simulink subsystem "ElectricalThermalSystemSSC"  (R2025b)
settings: Solver=VariableStepAuto  StartTime=0.0  StopTime=10.0  RelTol=1e-3
undefined symbols (not defined in the file): coolant_pipe_D, coolant_valve_D_ratio_max, coolant_valve_D_ratio_min, coolant_valve_displacement, EnvAirTemp, EnvGrvty, PlantThrEstCmpPwr, PlntThrChArea, PlntThrFanMaxSpd, PlntThrFanMechEff, PlntThrFanVolEff, PlntThrHeaterMaxPwr, PlntThrPipeArea, PlntThrPipeDia, PlntThrPmpMaxSpd, PlntThrRadRamEff, PlntThrRefrigAinit, PlntThrTankArea, PlntThrTankVol, PlntThrValDisp, PlntThrValDratioMax, PlntThrValDratioMin, PlntThrValSplMax, ThrmEM1, ThrmEM2, ThrmEM3, ThrmEM4
libraries: fl_lib x159, nesl_utility x69, SimscapeFluids_lib x25, autolibutils x12
(part 3 of 5)

== system ElectricalThermalSystemSSC/Battery/SC2 ==
  Absolute Reference (TL) : fl_lib/Thermal Liquid/Elements/Absolute Reference (TL)
  Mass & Energy Flow Rate Sensor (TL) : fl_lib/Thermal Liquid/Sensors/Flow Rate Sensor (TL)  mass_flow_measure=true  volumetric_flow_measure=false  energy_flow_measure=true
      settings: InternalSimscapePortConfiguration="{\"Bottom\":[{\"id\":\"PHI\",\"label\":\"φ\",\"type\":\"output\"}],\"Left\":[{\"id\":\"A\",\"label\":\"A\",\"type\":\"foundation.thermal_liquid.thermal_liquid\"}],\"Right\":[{\"id\":\"B\",\"label\":\"B\",\"type\":\"foundation.thermal_liquid.thermal_liquid\"},{\"id\":\"M\",\"label\":\"M\",\"type\":\"output\"}],\"Top\":[]}"
  PS-Simulink Converter : nesl_utility/PS-Simulink Converter  PhysicalDomain=network_engine_domain  SubClassName=ps_output  LeftPortType=input  RightPortType=output  PseudoPeriodic=off  Frequencies=[]  VectorFormat=1-D array  Unit=kg/s  AffineConversion=off
  Pressure & Temperature Sensor (TL) : fl_lib/Thermal Liquid/Sensors/Pressure & Temperature Sensor (TL)  reference=foundation.enum.MeasurementReference.difference  pressure=true  pressure_spec=foundation.enum.PressureMeasementSpec.Absolute  temperature=true
      settings: InternalSimscapePortConfiguration="{\"Bottom\":[{\"id\":\"T\",\"label\":\"T\",\"type\":\"output\"}],\"Left\":[{\"id\":\"A\",\"label\":\"A\",\"type\":\"foundation.thermal_liquid.thermal_liquid\"}],\"Right\":[{\"id\":\"B\",\"label\":\"B\",\"type\":\"foundation.thermal_liquid.thermal_liquid\"},{\"id\":\"P\",\"label\":\"P\",\"type\":\"output\"}],\"Top\":[]}"
  B : PMIOPort  Side=Left
  A : PMIOPort  Port=2  Side=Right
  01 : Outport
  wires:
  PS-Simulink Converter/1 -> 01/1
  connections:
  Mass & Energy Flow Rate Sensor (TL)/RConn2 -- PS-Simulink Converter/LConn1
  Absolute Reference (TL)/LConn1 -- Pressure & Temperature Sensor (TL)/RConn1
  Mass & Energy Flow Rate Sensor (TL)/RConn1 -- B/RConn1
  Mass & Energy Flow Rate Sensor (TL)/LConn1 -- A/RConn1 -- Pressure & Temperature Sensor (TL)/LConn1

== system ElectricalThermalSystemSSC/Battery Pump/LPF with IC1 ==
  u : Inport
  Cont LPF IC : autolibutils/Cont LPF IC  wc=wc  aMode=1  dataType=off
  Initial Condition : Constant  Value=InitCond  SampleTime=-1
  y : Outport
  wires:
  Cont LPF IC/1 -> y/1
  u/1 -> Cont LPF IC/1
  Initial Condition/1 -> Cont LPF IC/2

== system ElectricalThermalSystemSSC/Chiller Bypass Valve/LPF with IC1 ==
  u : Inport
  Cont LPF IC : autolibutils/Cont LPF IC  wc=wc  aMode=1  dataType=off
  Initial Condition : Constant  Value=InitCond  SampleTime=-1
  y : Outport
  wires:
  Cont LPF IC/1 -> y/1
  u/1 -> Cont LPF IC/1
  Initial Condition/1 -> Cont LPF IC/2

== system ElectricalThermalSystemSSC/DCDC/SC1 ==
  Absolute Reference (TL) : fl_lib/Thermal Liquid/Elements/Absolute Reference (TL)
  Mass & Energy Flow Rate Sensor (TL) : fl_lib/Thermal Liquid/Sensors/Flow Rate Sensor (TL)  mass_flow_measure=true  volumetric_flow_measure=false  energy_flow_measure=true
      settings: InternalSimscapePortConfiguration="{\"Bottom\":[{\"id\":\"PHI\",\"label\":\"φ\",\"type\":\"output\"}],\"Left\":[{\"id\":\"A\",\"label\":\"A\",\"type\":\"foundation.thermal_liquid.thermal_liquid\"}],\"Right\":[{\"id\":\"B\",\"label\":\"B\",\"type\":\"foundation.thermal_liquid.thermal_liquid\"},{\"id\":\"M\",\"label\":\"M\",\"type\":\"output\"}],\"Top\":[]}"
  PS-Simulink Converter : nesl_utility/PS-Simulink Converter  PhysicalDomain=network_engine_domain  SubClassName=ps_output  LeftPortType=input  RightPortType=output  PseudoPeriodic=off  Frequencies=[]  VectorFormat=1-D array  Unit=W  AffineConversion=off
  PS-Simulink Converter1 : nesl_utility/PS-Simulink Converter  PhysicalDomain=network_engine_domain  SubClassName=ps_output  LeftPortType=input  RightPortType=output  PseudoPeriodic=off  Frequencies=[]  VectorFormat=inherit  Unit=kg/s  AffineConversion=off
  Pressure & Temperature Sensor (TL) : fl_lib/Thermal Liquid/Sensors/Pressure & Temperature Sensor (TL)  reference=foundation.enum.MeasurementReference.difference  pressure=true  pressure_spec=foundation.enum.PressureMeasementSpec.Absolute  temperature=true
      settings: InternalSimscapePortConfiguration="{\"Bottom\":[{\"id\":\"T\",\"label\":\"T\",\"type\":\"output\"}],\"Left\":[{\"id\":\"A\",\"label\":\"A\",\"type\":\"foundation.thermal_liquid.thermal_liquid\"}],\"Right\":[{\"id\":\"B\",\"label\":\"B\",\"type\":\"foundation.thermal_liquid.thermal_liquid\"},{\"id\":\"P\",\"label\":\"P\",\"type\":\"output\"}],\"Top\":[]}"
  Terminator : Terminator
  Terminator1 : Terminator
  B : PMIOPort  Side=Left
  A : PMIOPort  Port=2  Side=Right
  wires:
  PS-Simulink Converter1/1 -> Terminator1/1
  PS-Simulink Converter/1 -> Terminator/1
  connections:
  PS-Simulink Converter1/LConn1 -- Mass & Energy Flow Rate Sensor (TL)/RConn2
  Mass & Energy Flow Rate Sensor (TL)/RConn3 -- PS-Simulink Converter/LConn1
  Absolute Reference (TL)/LConn1 -- Pressure & Temperature Sensor (TL)/RConn1
  Mass & Energy Flow Rate Sensor (TL)/RConn1 -- B/RConn1
  Mass & Energy Flow Rate Sensor (TL)/LConn1 -- A/RConn1 -- Pressure & Temperature Sensor (TL)/LConn1

== system ElectricalThermalSystemSSC/DCDC/SC2 ==
  Absolute Reference (TL) : fl_lib/Thermal Liquid/Elements/Absolute Reference (TL)
  Mass & Energy Flow Rate Sensor (TL) : fl_lib/Thermal Liquid/Sensors/Flow Rate Sensor (TL)  mass_flow_measure=true  volumetric_flow_measure=false  energy_flow_measure=true
      settings: InternalSimscapePortConfiguration="{\"Bottom\":[{\"id\":\"PHI\",\"label\":\"φ\",\"type\":\"output\"}],\"Left\":[{\"id\":\"A\",\"label\":\"A\",\"type\":\"foundation.thermal_liquid.thermal_liquid\"}],\"Right\":[{\"id\":\"B\",\"label\":\"B\",\"type\":\"foundation.thermal_liquid.thermal_liquid\"},{\"id\":\"M\",\"label\":\"M\",\"type\":\"output\"}],\"Top\":[]}"
  PS-Simulink Converter : nesl_utility/PS-Simulink Converter  PhysicalDomain=network_engine_domain  SubClassName=ps_output  LeftPortType=input  RightPortType=output  PseudoPeriodic=off  Frequencies=[]  VectorFormat=1-D array  Unit=W  AffineConversion=off
  Pressure & Temperature Sensor (TL) : fl_lib/Thermal Liquid/Sensors/Pressure & Temperature Sensor (TL)  reference=foundation.enum.MeasurementReference.difference  pressure=true  pressure_spec=foundation.enum.PressureMeasementSpec.Absolute  temperature=true
      settings: InternalSimscapePortConfiguration="{\"Bottom\":[{\"id\":\"T\",\"label\":\"T\",\"type\":\"output\"}],\"Left\":[{\"id\":\"A\",\"label\":\"A\",\"type\":\"foundation.thermal_liquid.thermal_liquid\"}],\"Right\":[{\"id\":\"B\",\"label\":\"B\",\"type\":\"foundation.thermal_liquid.thermal_liquid\"},{\"id\":\"P\",\"label\":\"P\",\"type\":\"output\"}],\"Top\":[]}"
  Terminator : Terminator
  B : PMIOPort  Side=Left
  A : PMIOPort  Port=2  Side=Right
  wires:
  PS-Simulink Converter/1 -> Terminator/1
  connections:
  Mass & Energy Flow Rate Sensor (TL)/RConn3 -- PS-Simulink Converter/LConn1
  Absolute Reference (TL)/LConn1 -- Pressure & Temperature Sensor (TL)/RConn1
  Mass & Energy Flow Rate Sensor (TL)/RConn1 -- B/RConn1
  Mass & Energy Flow Rate Sensor (TL)/LConn1 -- A/RConn1 -- Pressure & Temperature Sensor (TL)/LConn1

== system ElectricalThermalSystemSSC/Heater/LPF with IC1 ==
  u : Inport
  Cont LPF IC : autolibutils/Cont LPF IC  wc=wc  aMode=1  dataType=off
  Initial Condition : Constant  Value=InitCond  SampleTime=-1
  y : Outport
  wires:
  Cont LPF IC/1 -> y/1
  u/1 -> Cont LPF IC/1
  Initial Condition/1 -> Cont LPF IC/2

== system ElectricalThermalSystemSSC/Heater/SC1 ==
  Absolute Reference (TL) : fl_lib/Thermal Liquid/Elements/Absolute Reference (TL)
  Mass & Energy Flow Rate Sensor (TL) : fl_lib/Thermal Liquid/Sensors/Flow Rate Sensor (TL)  mass_flow_measure=true  volumetric_flow_measure=false  energy_flow_measure=true
      settings: InternalSimscapePortConfiguration="{\"Bottom\":[{\"id\":\"PHI\",\"label\":\"φ\",\"type\":\"output\"}],\"Left\":[{\"id\":\"A\",\"label\":\"A\",\"type\":\"foundation.thermal_liquid.thermal_liquid\"}],\"Right\":[{\"id\":\"B\",\"label\":\"B\",\"type\":\"foundation.thermal_liquid.thermal_liquid\"},{\"id\":\"M\",\"label\":\"M\",\"type\":\"output\"}],\"Top\":[]}"
  PS-Simulink Converter : nesl_utility/PS-Simulink Converter  PhysicalDomain=network_engine_domain  SubClassName=ps_output  LeftPortType=input  RightPortType=output  PseudoPeriodic=off  Frequencies=[]  VectorFormat=1-D array  Unit=W  AffineConversion=off
  PS-Simulink Converter1 : nesl_utility/PS-Simulink Converter  PhysicalDomain=network_engine_domain  SubClassName=ps_output  LeftPortType=input  RightPortType=output  PseudoPeriodic=off  Frequencies=[]  VectorFormat=inherit  Unit=K  AffineConversion=on
  Pressure & Temperature Sensor (TL) : fl_lib/Thermal Liquid/Sensors/Pressure & Temperature Sensor (TL)  reference=foundation.enum.MeasurementReference.difference  pressure=true  pressure_spec=foundation.enum.PressureMeasementSpec.Absolute  temperature=true
      settings: InternalSimscapePortConfiguration="{\"Bottom\":[{\"id\":\"T\",\"label\":\"T\",\"type\":\"output\"}],\"Left\":[{\"id\":\"A\",\"label\":\"A\",\"type\":\"foundation.thermal_liquid.thermal_liquid\"}],\"Right\":[{\"id\":\"B\",\"label\":\"B\",\"type\":\"foundation.thermal_liquid.thermal_liquid\"},{\"id\":\"P\",\"label\":\"P\",\"type\":\"output\"}],\"Top\":[]}"
  Terminator : Terminator
  Terminator1 : Terminator
  B : PMIOPort  Side=Left
  A : PMIOPort  Port=2  Side=Right
  wires:
  PS-Simulink Converter1/1 -> Terminator1/1
  PS-Simulink Converter/1 -> Terminator/1
  connections:
  PS-Simulink Converter1/LConn1 -- Pressure & Temperature Sensor (TL)/RConn3
  Mass & Energy Flow Rate Sensor (TL)/RConn3 -- PS-Simulink Converter/LConn1
  Absolute Reference (TL)/LConn1 -- Pressure & Temperature Sensor (TL)/RConn1
  Mass & Energy Flow Rate Sensor (TL)/RConn1 -- B/RConn1
  Mass & Energy Flow Rate Sensor (TL)/LConn1 -- A/RConn1 -- Pressure & Temperature Sensor (TL)/LConn1

== system ElectricalThermalSystemSSC/Heater/SC2 ==
  Absolute Reference (TL) : fl_lib/Thermal Liquid/Elements/Absolute Reference (TL)
  Mass & Energy Flow Rate Sensor (TL) : fl_lib/Thermal Liquid/Sensors/Flow Rate Sensor (TL)  mass_flow_measure=true  volumetric_flow_measure=false  energy_flow_measure=true
      settings: InternalSimscapePortConfiguration="{\"Bottom\":[{\"id\":\"PHI\",\"label\":\"φ\",\"type\":\"output\"}],\"Left\":[{\"id\":\"A\",\"label\":\"A\",\"type\":\"foundation.thermal_liquid.thermal_liquid\"}],\"Right\":[{\"id\":\"B\",\"label\":\"B\",\"type\":\"foundation.thermal_liquid.thermal_liquid\"},{\"id\":\"M\",\"label\":\"M\",\"type\":\"output\"}],\"Top\":[]}"
  PS-Simulink Converter : nesl_utility/PS-Simulink Converter  PhysicalDomain=network_engine_domain  SubClassName=ps_output  LeftPortType=input  RightPortType=output  PseudoPeriodic=off  Frequencies=[]  VectorFormat=1-D array  Unit=W  AffineConversion=off
  Pressure & Temperature Sensor (TL) : fl_lib/Thermal Liquid/Sensors/Pressure & Temperature Sensor (TL)  reference=foundation.enum.MeasurementReference.difference  pressure=true  pressure_spec=foundation.enum.PressureMeasementSpec.Absolute  temperature=true
      settings: InternalSimscapePortConfiguration="{\"Bottom\":[{\"id\":\"T\",\"label\":\"T\",\"type\":\"output\"}],\"Left\":[{\"id\":\"A\",\"label\":\"A\",\"type\":\"foundation.thermal_liquid.thermal_liquid\"}],\"Right\":[{\"id\":\"B\",\"label\":\"B\",\"type\":\"foundation.thermal_liquid.thermal_liquid\"},{\"id\":\"P\",\"label\":\"P\",\"type\":\"output\"}],\"Top\":[]}"
  Terminator : Terminator
  B : PMIOPort  Side=Left
  A : PMIOPort  Port=2  Side=Right
  wires:
  PS-Simulink Converter/1 -> Terminator/1
  connections:
  Mass & Energy Flow Rate Sensor (TL)/RConn3 -- PS-Simulink Converter/LConn1
  Absolute Reference (TL)/LConn1 -- Pressure & Temperature Sensor (TL)/RConn1
  Mass & Energy Flow Rate Sensor (TL)/RConn1 -- B/RConn1
  Mass & Energy Flow Rate Sensor (TL)/LConn1 -- A/RConn1 -- Pressure & Temperature Sensor (TL)/LConn1

== system ElectricalThermalSystemSSC/Motor/Cooling Assembly ==
  CoolingAssy1 : Subsystem  VariantControl=PlntEMNum == 1
  CoolingAssy2 : Subsystem  VariantControl=PlntEMNum == 2
  CoolingAssy3 : Subsystem  VariantControl=PlntEMNum == 3
  CoolingAssy4 : Subsystem  VariantControl=PlntEMNum == 4
  A : PMIOPort  Side=Left
  B : PMIOPort  Port=2  Side=Right
  H4 : PMIOPort  Port=3  Side=Right
  H3 : PMIOPort  Port=4  Side=Right
  H2 : PMIOPort  Port=5  Side=Right
  H1 : PMIOPort  Port=6  Side=Right
  EMTemp : Outport
  Qem : Outport  Port=2

== system ElectricalThermalSystemSSC/Motor Pump/LPF with IC1 ==
  u : Inport
  Cont LPF IC : autolibutils/Cont LPF IC  wc=wc  aMode=1  dataType=off
  Initial Condition : Constant  Value=InitCond  SampleTime=-1
  y : Outport
  wires:
  Cont LPF IC/1 -> y/1
  u/1 -> Cont LPF IC/1
  Initial Condition/1 -> Cont LPF IC/2

== system ElectricalThermalSystemSSC/Parallel-Serial Mode Valve/Battery Coolant Tank Heat Transfer ==
  AmbTemp : Inport
  Convective Heat Transfer : fl_lib/Thermal/Thermal Elements/Convective Heat Transfer  thermal_type=foundation.enum.constant_variable.constant  area=3 * PlntThrTankArea m^2  heat_tr_coeff=20 W/(m^2 * K)  min_heat_tr_coeff=1e-3 W/(K*m^2)  T_specify=off  T_priority=None  T=0 K  T_nominal_specify=off  T_nominal_value=1  T_nominal_unit=K  Q_specify=off  Q_priority=None  Q=0 W  Q_nominal_specify=off  Q_nominal_value=1  Q_nominal_unit=W
  Convective Heat Transfer1 : fl_lib/Thermal/Thermal Elements/Convective Heat Transfer  thermal_type=foundation.enum.constant_variable.constant  area=3 * PlntThrTankArea m^2  heat_tr_coeff=20 W/(m^2 * K)  min_heat_tr_coeff=1e-3 W/(K*m^2)  T_specify=off  T_priority=None  T=0 K  T_nominal_specify=off  T_nominal_value=1  T_nominal_unit=K  Q_specify=off  Q_priority=None  Q=0 W  Q_nominal_specify=off  Q_nominal_value=1  Q_nominal_unit=W
  Environment Temperature : fl_lib/Thermal/Thermal Sources/Controlled Temperature Source
  Simulink-PS Converter : nesl_utility/Simulink-PS Converter  PhysicalDomain=network_engine_domain  SubClassName=ps_input  LeftPortType=input  RightPortType=output  PseudoPeriodic=off  Frequencies=[]  NoiseDistribution=none  NoiseParameters=[]  Unit=K  AffineConversion=on  FilteringAndDerivatives=provide  SimscapeFilterOrder=1  InputFilterTimeConstant=0.001  UdotUserProvided=0
  Thermal Reference : fl_lib/Thermal/Thermal Elements/Thermal Reference
  A : PMIOPort  Side=Left
  B : PMIOPort  Port=2  Side=Left
  wires:
  AmbTemp/1 -> Simulink-PS Converter/1
  connections:
  Convective Heat Transfer/LConn1 -- A/RConn1
  B/RConn1 -- Convective Heat Transfer1/LConn1
  Simulink-PS Converter/RConn1 -- Environment Temperature/RConn1
  Thermal Reference/LConn1 -- Environment Temperature/RConn2
  Convective Heat Transfer1/RConn1 -- Convective Heat Transfer/RConn1 -- Environment Temperature/LConn1

== system ElectricalThermalSystemSSC/Parallel-Serial Mode Valve/LPF with IC1 ==
  u : Inport
  Cont LPF IC : autolibutils/Cont LPF IC  wc=wc  aMode=1  dataType=off
  Initial Condition : Constant  Value=InitCond  SampleTime=-1
  y : Outport
  wires:
  Cont LPF IC/1 -> y/1
  u/1 -> Cont LPF IC/1
  Initial Condition/1 -> Cont LPF IC/2

== system ElectricalThermalSystemSSC/Parallel-Serial Mode Valve/Motor Coolant Tank Heat Transfer ==
  AmbTemp : Inport
  Convective Heat Transfer : fl_lib/Thermal/Thermal Elements/Convective Heat Transfer  thermal_type=foundation.enum.constant_variable.constant  area=3 * PlntThrTankArea m^2  heat_tr_coeff=20 W/(m^2 * K)  min_heat_tr_coeff=1e-3 W/(K*m^2)  T_specify=off  T_priority=None  T=0 K  T_nominal_specify=off  T_nominal_value=1  T_nominal_unit=K  Q_specify=off  Q_priority=None  Q=0 W  Q_nominal_specify=off  Q_nominal_value=1  Q_nominal_unit=W
  Convective Heat Transfer1 : fl_lib/Thermal/Thermal Elements/Convective Heat Transfer  thermal_type=foundation.enum.constant_variable.constant  area=3 * PlntThrTankArea m^2  heat_tr_coeff=20 W/(m^2 * K)  min_heat_tr_coeff=1e-3 W/(K*m^2)  T_specify=off  T_priority=None  T=0 K  T_nominal_specify=off  T_nominal_value=1  T_nominal_unit=K  Q_specify=off  Q_priority=None  Q=0 W  Q_nominal_specify=off  Q_nominal_value=1  Q_nominal_unit=W
  Environment Temperature : fl_lib/Thermal/Thermal Sources/Controlled Temperature Source
  Simulink-PS Converter : nesl_utility/Simulink-PS Converter  PhysicalDomain=network_engine_domain  SubClassName=ps_input  LeftPortType=input  RightPortType=output  PseudoPeriodic=off  Frequencies=[]  NoiseDistribution=none  NoiseParameters=[]  Unit=K  AffineConversion=on  FilteringAndDerivatives=provide  SimscapeFilterOrder=1  InputFilterTimeConstant=0.001  UdotUserProvided=0
  Thermal Reference : fl_lib/Thermal/Thermal Elements/Thermal Reference
  A : PMIOPort  Side=Right
  B : PMIOPort  Port=2  Side=Right
  wires:
  AmbTemp/1 -> Simulink-PS Converter/1
  connections:
  A/RConn1 -- Convective Heat Transfer/LConn1
  B/RConn1 -- Convective Heat Transfer1/LConn1
  Convective Heat Transfer1/RConn1 -- Environment Temperature/LConn1 -- Convective Heat Transfer/RConn1
  Thermal Reference/LConn1 -- Environment Temperature/RConn2
  Simulink-PS Converter/RConn1 -- Environment Temperature/RConn1

== system ElectricalThermalSystemSSC/Radiator/Ram Pressure ==
  1/2 : fl_lib/Physical Signals/Functions/PS Gain  gain=0.5
  Controlled Pressure Source (MA) : fl_lib/Moist Air/Sources/Pressure Source (MA)  source_type=foundation.enum.constant_controlled.controlled  pressure_differential=0 MPa  power_spec=foundation.enum.power_spec.isentropic  area_A=PlntThrCabDucArea m^2  area_B=PlntThrCabDucArea m^2
      settings: InternalSimscapePortConfiguration="{\"Bottom\":[],\"Left\":[{\"id\":\"A\",\"label\":\"A\",\"type\":\"foundation.moist_air.moist_air\"},{\"id\":\"P\",\"label\":\"P\",\"type\":\"input\"}],\"Right\":[{\"id\":\"B\",\"label\":\"B\",\"type\":\"foundation.moist_air.moist_air\"}],\"Top\":[]}"
  PS Gain : fl_lib/Physical Signals/Functions/PS Gain  gain=PlntThrRadRamEff
  PS Product : fl_lib/Physical Signals/Functions/PS Product
  Thermodynamic Properties Sensor (MA) : fl_lib/Moist Air/Sensors/Thermodynamic Properties Sensor (MA)  measurement_mass_spec=foundation.enum.measurement_mass_spec.mixture  enthalpy=true  enthalpy_reference=foundation.enum.EnthalpyReference.PropertyTables  density=true  specific_heat=true  entropy=true
      settings: InternalSimscapePortConfiguration="{\"Bottom\":[{\"id\":\"CP\",\"label\":\"cp\",\"type\":\"output\"},{\"id\":\"S\",\"label\":\"s\",\"type\":\"output\"}],\"Left\":[{\"id\":\"A\",\"label\":\"A\",\"type\":\"foundation.moist_air.moist_air\"}],\"Right\":[{\"id\":\"H\",\"label\":\"h\",\"type\":\"output\"},{\"id\":\"RHO\",\"label\":\"ρ\",\"type\":\"output\"}],\"Top\":[]}"
  sqr : fl_lib/Physical Signals/Functions/PS Math Function  fcn_choice=foundation.enum.math_function.square  v=1
  A : PMIOPort  Side=Left
  V : PMIOPort  Port=2  Side=Left
  B : PMIOPort  Port=3  Side=Right
  connections:
  Thermodynamic Properties Sensor (MA)/RConn2 -- PS Product/LConn2
  V/RConn1 -- sqr/LConn1
  sqr/RConn1 -- 1/2/LConn1
  1/2/RConn1 -- PS Gain/LConn1
  PS Product/RConn1 -- Controlled Pressure Source (MA)/LConn2
  Thermodynamic Properties Sensor (MA)/LConn1 -- A/RConn1 -- Controlled Pressure Source (MA)/LConn1
  Controlled Pressure Source (MA)/RConn1 -- B/RConn1
  PS Gain/RConn1 -- PS Product/LConn1

== system ElectricalThermalSystemSSC/Radiator/SC1 ==
  Absolute Reference (TL) : fl_lib/Thermal Liquid/Elements/Absolute Reference (TL)
  Mass & Energy Flow Rate Sensor (TL) : fl_lib/Thermal Liquid/Sensors/Flow Rate Sensor (TL)  mass_flow_measure=true  volumetric_flow_measure=false  energy_flow_measure=true
      settings: InternalSimscapePortConfiguration="{\"Bottom\":[{\"id\":\"PHI\",\"label\":\"φ\",\"type\":\"output\"}],\"Left\":[{\"id\":\"A\",\"label\":\"A\",\"type\":\"foundation.thermal_liquid.thermal_liquid\"}],\"Right\":[{\"id\":\"B\",\"label\":\"B\",\"type\":\"foundation.thermal_liquid.thermal_liquid\"},{\"id\":\"M\",\"label\":\"M\",\"type\":\"output\"}],\"Top\":[]}"
  PS-Simulink Converter1 : nesl_utility/PS-Simulink Converter  PhysicalDomain=network_engine_domain  SubClassName=ps_output  LeftPortType=input  RightPortType=output  PseudoPeriodic=off  Frequencies=[]  VectorFormat=inherit  Unit=K  AffineConversion=on
  Pressure & Temperature Sensor (TL) : fl_lib/Thermal Liquid/Sensors/Pressure & Temperature Sensor (TL)  reference=foundation.enum.MeasurementReference.difference  pressure=true  pressure_spec=foundation.enum.PressureMeasementSpec.Absolute  temperature=true
      settings: InternalSimscapePortConfiguration="{\"Bottom\":[{\"id\":\"T\",\"label\":\"T\",\"type\":\"output\"}],\"Left\":[{\"id\":\"A\",\"label\":\"A\",\"type\":\"foundation.thermal_liquid.thermal_liquid\"}],\"Right\":[{\"id\":\"B\",\"label\":\"B\",\"type\":\"foundation.thermal_liquid.thermal_liquid\"},{\"id\":\"P\",\"label\":\"P\",\"type\":\"output\"}],\"Top\":[]}"
  Terminator1 : Terminator
  B : PMIOPort  Side=Left
  A : PMIOPort  Port=2  Side=Right
  RadIn : PMIOPort  Port=3  Side=Left
  wires:
  PS-Simulink Converter1/1 -> Terminator1/1
  connections:
  RadIn/RConn1 -- Mass & Energy Flow Rate Sensor (TL)/RConn3
  Absolute Reference (TL)/LConn1 -- Pressure & Temperature Sensor (TL)/RConn1
  Mass & Energy Flow Rate Sensor (TL)/RConn1 -- B/RConn1
  Mass & Energy Flow Rate Sensor (TL)/LConn1 -- A/RConn1 -- Pressure & Temperature Sensor (TL)/LConn1
  PS-Simulink Converter1/LConn1 -- Pressure & Temperature Sensor (TL)/RConn3

== system ElectricalThermalSystemSSC/Radiator/SC2 ==
  Absolute Reference (TL) : fl_lib/Thermal Liquid/Elements/Absolute Reference (TL)
  Mass & Energy Flow Rate Sensor (TL) : fl_lib/Thermal Liquid/Sensors/Flow Rate Sensor (TL)  mass_flow_measure=true  volumetric_flow_measure=false  energy_flow_measure=true
      settings: InternalSimscapePortConfiguration="{\"Bottom\":[{\"id\":\"PHI\",\"label\":\"φ\",\"type\":\"output\"}],\"Left\":[{\"id\":\"A\",\"label\":\"A\",\"type\":\"foundation.thermal_liquid.thermal_liquid\"}],\"Right\":[{\"id\":\"B\",\"label\":\"B\",\"type\":\"foundation.thermal_liquid.thermal_liquid\"},{\"id\":\"M\",\"label\":\"M\",\"type\":\"output\"}],\"Top\":[]}"
  PS-Simulink Converter1 : nesl_utility/PS-Simulink Converter  PhysicalDomain=network_engine_domain  SubClassName=ps_output  LeftPortType=input  RightPortType=output  PseudoPeriodic=off  Frequencies=[]  VectorFormat=inherit  Unit=K  AffineConversion=on
  Pressure & Temperature Sensor (TL) : fl_lib/Thermal Liquid/Sensors/Pressure & Temperature Sensor (TL)  reference=foundation.enum.MeasurementReference.difference  pressure=true  pressure_spec=foundation.enum.PressureMeasementSpec.Absolute  temperature=true
      settings: InternalSimscapePortConfiguration="{\"Bottom\":[{\"id\":\"T\",\"label\":\"T\",\"type\":\"output\"}],\"Left\":[{\"id\":\"A\",\"label\":\"A\",\"type\":\"foundation.thermal_liquid.thermal_liquid\"}],\"Right\":[{\"id\":\"B\",\"label\":\"B\",\"type\":\"foundation.thermal_liquid.thermal_liquid\"},{\"id\":\"P\",\"label\":\"P\",\"type\":\"output\"}],\"Top\":[]}"
  Terminator1 : Terminator
  B : PMIOPort  Side=Left
  A : PMIOPort  Port=2  Side=Right
  RadOut : PMIOPort  Port=3  Side=Left
  wires:
  PS-Simulink Converter1/1 -> Terminator1/1
  connections:
  Absolute Reference (TL)/LConn1 -- Pressure & Temperature Sensor (TL)/RConn1
  Mass & Energy Flow Rate Sensor (TL)/RConn1 -- B/RConn1
  Mass & Energy Flow Rate Sensor (TL)/LConn1 -- A/RConn1 -- Pressure & Temperature Sensor (TL)/LConn1
  PS-Simulink Converter1/LConn1 -- Pressure & Temperature Sensor (TL)/RConn3
  RadOut/RConn1 -- Mass & Energy Flow Rate Sensor (TL)/RConn3

== system ElectricalThermalSystemSSC/Radiator Bypass Valve/LPF with IC1 ==
  u : Inport
  Cont LPF IC : autolibutils/Cont LPF IC  wc=wc  aMode=1  dataType=off
  Initial Condition : Constant  Value=InitCond  SampleTime=-1
  y : Outport
  wires:
  Cont LPF IC/1 -> y/1
  u/1 -> Cont LPF IC/1
  Initial Condition/1 -> Cont LPF IC/2

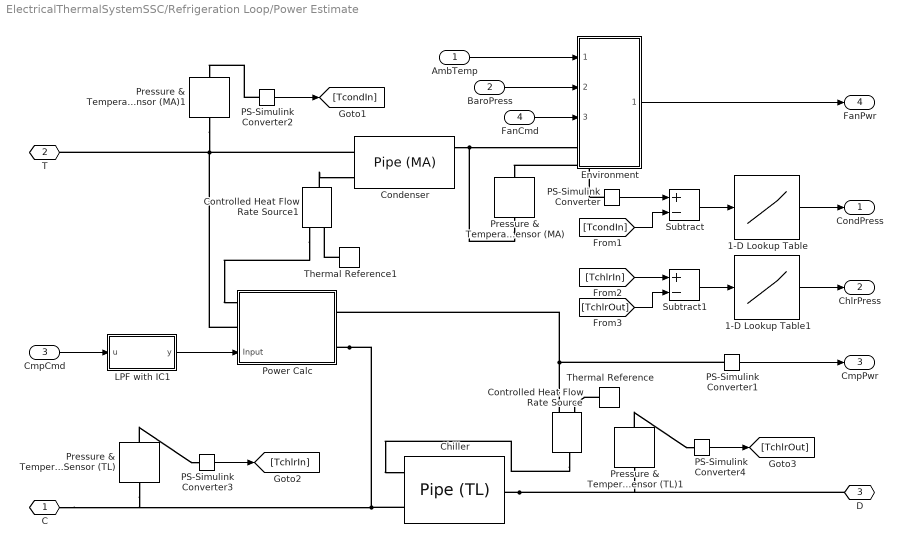
== system ElectricalThermalSystemSSC/Refrigeration Loop/Power Estimate ==
  AmbTemp : Inport
  BaroPress : Inport  Port=2
  CmpCmd : Inport  Port=3
  FanCmd : Inport  Port=4
  1-D Lookup Table : Lookup_n-D  NumberOfTableDimensions=1  BreakpointsForDimension1=[0 4.5 10 13 20]  Table=[1.3 1.3 1.53 1.62 1.7]  ExtrapMethod=Clip  UseLastTableValue=on  InternalRulePriority=Speed  RndMeth=Simplest
  1-D Lookup Table1 : Lookup_n-D  NumberOfTableDimensions=1  BreakpointsForDimension1=[0 1 3 7]  Table=[0.65 0.45 0.3 0.3]  ExtrapMethod=Clip  UseLastTableValue=on  InternalRulePriority=Speed  RndMeth=Simplest
  Chiller : fl_lib/Thermal Liquid/Elements/Pipe (TL)  length=1 m  area=PlntThrPipeArea m^2  Dh=PlntThrPipeDia m  length_add=0.1 m  roughness=15e-6 m  Re_lam=2000  Re_tur=4000  shape_factor=64  Nu_lam=3.66  dynamic_compressibility=simscape.enum.onoff.on  inertia=simscape.enum.onoff.off  p0=EnvAbsPrs Pa  T0=EnvAirTemp K  mdot0=0 kg/s  p_nominal=0.101325 MPa  T_nominal=293.15 K
  Condenser : fl_lib/Moist Air/Elements/Pipe (MA)  length=0.5 m  area=PlntThrCabDucArea m^2  Dh=PlntThrCabHydDia m  length_add=0 m  roughness=15e-6 m  Re_lam=2000  Re_tur=4000  shape_factor=64  Nu_lam=3.66  wall_condensation=simscape.enum.onoff.off  RH_ws=1  time_constant_cond=1e-3 s  time_constant_evap=1e-3 s  fraction_entrained=1  moisture_trace_gas_source=foundation.enum.moisture_trace_gas_source.none  moisture_source_spec=foundation.enum.MoistureSourceSpec.WaterVapor  vapor_from_liquid=false  moisture_mass_flow=0 kg/s  moisture_temperature_spec=foundation.enum.temperature_spec.atmospheric  moisture_temperature=293.15 K  trace_gas_mass_flow=0 kg/s  trace_gas_temperature_spec=foundation.enum.temperature_spec.atmospheric  trace_gas_temperature=293.15 K  p_init=EnvAbsPrs Pa  p_init_priority=foundation.enum.Priority.High  T_init=EnvAirTemp K  T_init_priority=foundation.enum.Priority.High  humidity_spec=foundation.enum.HumiditySpec.RelativeHumidity  RH_init=PlntThrCabRelHInit  RH_init_priority=foundation.enum.Priority.High  x_w_init=0  x_w_init_priority=foundation.enum.Priority.None  y_w_init=0  y_w_init_priority=foundation.enum.Priority.None  HR_init=0  HR_init_priority=foundation.enum.Priority.None  Tw_init=287 K  Tw_init_priority=foundation.enum.Priority.High  trace_gas_spec=foundation.enum.trace_gas_spec.mole_fraction  x_g_init=0  x_g_init_priority=foundation.enum.Priority.None  y_g_init=PlntThrCabCO2Init  y_g_init_priority=foundation.enum.Priority.High  r_d_init=0  r_d_init_priority=foundation.enum.Priority.High
  Controlled Heat Flow Rate Source : fl_lib/Thermal/Thermal Sources/Controlled Heat Flow Rate Source
  Controlled Heat Flow Rate Source1 : fl_lib/Thermal/Thermal Sources/Controlled Heat Flow Rate Source
  Environment : Subsystem
  LPF with IC1 : Subsystem  mask{wc=0.2, InitCond=0, dataType=off}
      mask prompts: wc "Cutoff frequency, wc [rad/s]"; InitCond "Initial condition, InitCond [same as u]"; dataType "Enforce same input data type"
      mask TypeOptions wc: Cont LPF IC/wc
      mask TypeOptions InitCond: Initial Condition/Value
      mask TypeOptions dataType: Cont LPF IC/dataType
  PS-Simulink Converter{,2..4} (4 alike) : nesl_utility/PS-Simulink Converter  PhysicalDomain=network_engine_domain  SubClassName=ps_output  LeftPortType=input  RightPortType=output  PseudoPeriodic=off  Frequencies=[]  VectorFormat=inherit  Unit=inherit  AffineConversion=off
  PS-Simulink Converter1 : nesl_utility/PS-Simulink Converter  PhysicalDomain=network_engine_domain  SubClassName=ps_output  LeftPortType=input  RightPortType=output  PseudoPeriodic=off  Frequencies=[]  VectorFormat=inherit  Unit=W  AffineConversion=off
  Power Calc : Subsystem
      settings: PortSchema="{\"entries\":[{\"content\":{\"sides\":[{\"content\":{\"connectorIds\":[\"LConn1\",\"LConn2\",\"In1\"]},\"type\":\"ConnectorPlacement.EquallySpacedRectSide\",\"uuid\":\"d10d0531-d19f-4f48-9498-1b632de709af\"},{\"content\":{\"connectorIds\":[\"RConn1\",\"RConn2\"],\"side\":\"RIGHT\"},\"type\":\"ConnectorPlacement.EquallySpacedRectSide\",\"uuid\":\"2d98f368-42ce-45c2-8dbe-64480dd2dfe3\"},{\"content\":{\"side\":\"TOP\"},\"type\":\"ConnectorPlacement.EquallySpacedRectSide\",\"uuid\":\"0326b993-af28-4eca-ba8b-7a5fc9524b87\"}]},\"type\":\"ConnectorPlacement.EquallySpacedConnector\",\"uuid\":\"886ec53b-5c74-488a-b138-2ba602235742\"}],\"packageUris\":[\"http://schema.mathworks.com/mf0/Connector/R2020b\"],\"version\":\"1.0\"}"
  Pressure & Temperature Sensor (MA) : fl_lib/Moist Air/Sensors/Pressure & Temperature Sensor (MA)  reference=foundation.enum.MeasurementReference.absolute  pressure=false  pressure_spec=foundation.enum.PressureMeasementSpec.Absolute  temperature=true
      settings: InternalSimscapePortConfiguration="{\"Bottom\":[{\"id\":\"T\",\"label\":\"T\",\"type\":\"output\"}],\"Left\":[{\"id\":\"A\",\"label\":\"A\",\"type\":\"foundation.moist_air.moist_air\"}],\"Right\":[],\"Top\":[]}"
  Pressure & Temperature Sensor (MA)1 : fl_lib/Moist Air/Sensors/Pressure & Temperature Sensor (MA)  reference=foundation.enum.MeasurementReference.absolute  pressure=false  pressure_spec=foundation.enum.PressureMeasementSpec.Absolute  temperature=true
      settings: InternalSimscapePortConfiguration="{\"Bottom\":[{\"id\":\"T\",\"label\":\"T\",\"type\":\"output\"}],\"Left\":[{\"id\":\"A\",\"label\":\"A\",\"type\":\"foundation.moist_air.moist_air\"}],\"Right\":[],\"Top\":[]}"
  Pressure & Temperature Sensor (TL) : fl_lib/Thermal Liquid/Sensors/Pressure & Temperature Sensor (TL)  reference=foundation.enum.MeasurementReference.absolute  pressure=false  pressure_spec=foundation.enum.PressureMeasementSpec.Absolute  temperature=true
      settings: InternalSimscapePortConfiguration="{\"Bottom\":[{\"id\":\"T\",\"label\":\"T\",\"type\":\"output\"}],\"Left\":[{\"id\":\"A\",\"label\":\"A\",\"type\":\"foundation.thermal_liquid.thermal_liquid\"}],\"Right\":[],\"Top\":[]}"
  Pressure & Temperature Sensor (TL)1 : fl_lib/Thermal Liquid/Sensors/Pressure & Temperature Sensor (TL)  reference=foundation.enum.MeasurementReference.absolute  pressure=false  pressure_spec=foundation.enum.PressureMeasementSpec.Absolute  temperature=true
      settings: InternalSimscapePortConfiguration="{\"Bottom\":[{\"id\":\"T\",\"label\":\"T\",\"type\":\"output\"}],\"Left\":[{\"id\":\"A\",\"label\":\"A\",\"type\":\"foundation.thermal_liquid.thermal_liquid\"}],\"Right\":[],\"Top\":[]}"
  Subtract : Sum  Inputs=+-
  Subtract1 : Sum  Inputs=+-
  Thermal Reference : fl_lib/Thermal/Thermal Elements/Thermal Reference
  Thermal Reference1 : fl_lib/Thermal/Thermal Elements/Thermal Reference
  C : PMIOPort  Side=Left
  T : PMIOPort  Port=2  Side=Left
  D : PMIOPort  Port=3  Side=Right
  CondPress : Outport
  ChlrPress : Outport  Port=2
  CmpPwr : Outport  Port=3
  FanPwr : Outport  Port=4
  wires:
  1-D Lookup Table1/1 -> ChlrPress/1
  1-D Lookup Table/1 -> CondPress/1
  [TchlrIn] -> Subtract1/1
  [TcondIn] -> Subtract/2
  [TchlrOut] -> Subtract1/2
  PS-Simulink Converter/1 -> Subtract/1
  Subtract1/1 -> 1-D Lookup Table1/1
  Subtract/1 -> 1-D Lookup Table/1
  PS-Simulink Converter2/1 -> [TcondIn]
  PS-Simulink Converter3/1 -> [TchlrIn]
  PS-Simulink Converter4/1 -> [TchlrOut]
  LPF with IC1/1(y) -> Power Calc/1(Input)
  CmpCmd/1 -> LPF with IC1/1(u)
  AmbTemp/1 -> Environment/1(AmbTemp)
  BaroPress/1 -> Environment/2(BaroPress)
  FanCmd/1 -> Environment/3(FanCmd)
  Environment/1(FanPwr) -> FanPwr/1
  PS-Simulink Converter1/1 -> CmpPwr/1
  connections:
  PS-Simulink Converter/LConn1 -- Pressure & Temperature Sensor (MA)/RConn1
  PS-Simulink Converter2/LConn1 -- Pressure & Temperature Sensor (MA)1/RConn1
  Pressure & Temperature Sensor (TL)/RConn1 -- PS-Simulink Converter3/LConn1
  Pressure & Temperature Sensor (TL)1/RConn1 -- PS-Simulink Converter4/LConn1
  Controlled Heat Flow Rate Source1/LConn1 -- Condenser/LConn2
  Thermal Reference1/LConn1 -- Controlled Heat Flow Rate Source1/RConn2
  Controlled Heat Flow Rate Source1/RConn1 -- Power Calc/LConn1
  PS-Simulink Converter1/LConn1 -- Power Calc/RConn1 -- Controlled Heat Flow Rate Source/RConn1
  Thermal Reference/LConn1 -- Controlled Heat Flow Rate Source/RConn2
  Controlled Heat Flow Rate Source/LConn1 -- Chiller/LConn2
  Power Calc/RConn2 -- Chiller/LConn1 -- Pressure & Temperature Sensor (TL)/LConn1 -- C/RConn1
  Pressure & Temperature Sensor (MA)1/LConn1 -- T/RConn1 -- Condenser/LConn1 -- Power Calc/LConn2
  Pressure & Temperature Sensor (MA)/LConn1 -- Environment/LConn1 -- Condenser/RConn1
  Chiller/RConn1 -- Pressure & Temperature Sensor (TL)1/LConn1 -- D/RConn1

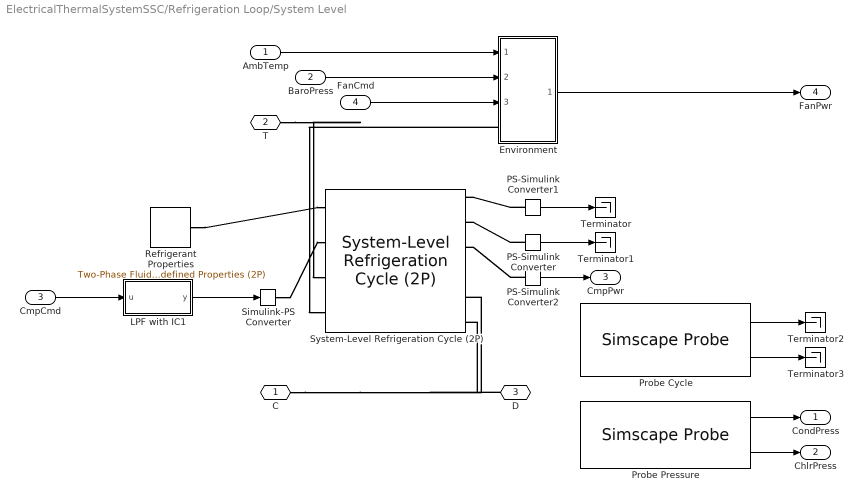
== system ElectricalThermalSystemSSC/Refrigeration Loop/System Level ==
  AmbTemp : Inport
  BaroPress : Inport  Port=2
  CmpCmd : Inport  Port=3
  FanCmd : Inport  Port=4
  Environment : Subsystem
  LPF with IC1 : Subsystem  mask{wc=0.2, InitCond=0, dataType=off}
      mask prompts: wc "Cutoff frequency, wc [rad/s]"; InitCond "Initial condition, InitCond [same as u]"; dataType "Enforce same input data type"
      mask TypeOptions wc: Cont LPF IC/wc
      mask TypeOptions InitCond: Initial Condition/Value
      mask TypeOptions dataType: Cont LPF IC/dataType
  PS-Simulink Converter : nesl_utility/PS-Simulink Converter  PhysicalDomain=network_engine_domain  SubClassName=ps_output  LeftPortType=input  RightPortType=output  PseudoPeriodic=off  Frequencies=[]  VectorFormat=inherit  Unit=W  AffineConversion=off
  PS-Simulink Converter1 : nesl_utility/PS-Simulink Converter  PhysicalDomain=network_engine_domain  SubClassName=ps_output  LeftPortType=input  RightPortType=output  PseudoPeriodic=off  Frequencies=[]  VectorFormat=inherit  Unit=W  AffineConversion=off
  PS-Simulink Converter2 : nesl_utility/PS-Simulink Converter  PhysicalDomain=network_engine_domain  SubClassName=ps_output  LeftPortType=input  RightPortType=output  PseudoPeriodic=off  Frequencies=[]  VectorFormat=inherit  Unit=W  AffineConversion=off
  Probe Cycle : SimscapeProbe  BoundBlock=25446  Variables={h_cycle, p_cycle}
  Probe Pressure : SimscapeProbe  BoundBlock=25446  Variables={condenser.refrigerant.p, evaporator.refrigerant.p}
  Refrigerant Properties : SimscapeFluids_lib/Two-Phase Fluid/Utilities/Two-Phase Fluid Predefined Properties (2P)  fluid=fluids.two_phase_fluid.utilities.enum.Fluid.R134a  p_atm=0.101325 MPa  properties_range_check=simscape.enum.assert.action.error  q_rev=0.01 Pa
  Simulink-PS Converter : nesl_utility/Simulink-PS Converter  PhysicalDomain=network_engine_domain  SubClassName=ps_input  LeftPortType=input  RightPortType=output  PseudoPeriodic=off  Frequencies=[]  NoiseDistribution=none  NoiseParameters=[]  Unit=1  AffineConversion=off  FilteringAndDerivatives=provide  SimscapeFilterOrder=1  InputFilterTimeConstant=0.001  UdotUserProvided=0
  System-Level Refrigeration Cycle (2P) : SimscapeFluids_lib/Two-Phase Fluid/Thermodynamic Cycles/System-Level Refrigeration Cycle (2P)  capacity_spec=fluids.two_phase_fluid.thermodynamic_cycles.enum.RefrigerationCycleCapacitySpec.CoolingLoad  Q_cond_nominal=15 kW  Q_evap_nominal=PlntThrCycNomHeatflw kW  mdot_nominal=0.005 kg/s  pressure_spec=fluids.two_phase_fluid.thermodynamic_cycles.enum.RefrigerationCyclePressureSpec.Pressure  p_cond_nominal=PlntThrCycCondRefPin kPa  p_evap_nominal=PlntThrCycChlrRefPin kPa  T_cond_nominal=333.15 K  T_evap_nominal=273.15 K  delta_T_sub_nominal=5 deltaK  delta_T_sup_nominal=10 deltaK  delta_T_sup_static=5 deltaK  performance_spec=fluids.two_phase_fluid.thermodynamic_cycles.enum.RefrigerationCyclePerformanceSpec.COPCooling  COP_nominal=3  comp_eta_s=0.8  comp_eta_v_nominal=0.95  comp_eta_m=0.95  valve_max_fraction=1.5  valve_leak_fraction=1e-6  valve_smoothing_factor=0.01  volume_cond=PlntThrCycCondRefVol m^3  volume_evap=PlntThrCycChlrRefVol m^3  receiver_volume=2 l  receiver_L_init=1 - PlntThrRefrigAinit  nominal_init=true  p_cond_init=refrigerant_p_init MPa  p_evap_init=refrigerant_p_init MPa  h_cond_init=[450, 250] kJ/kg  h_evap_init=[250, 400] kJ/kg  receiver_saturated_init=true  receiver_h_liq_init=500 kJ/kg  receiver_h_vap_init=3500 kJ/kg  cond_domain=fluids.two_phase_fluid.thermodynamic_cycles.enum.RefrigerationCycleFluidDomain.MoistAir  cond_mdot_nominal=PlntThrCycCondAirFlw kg/s  cond_delta_p_nominal=PlntThrCondNomAirDP Pa  cond_pressure_spec=fluids.two_phase_fluid.thermodynamic_cycles.enum.RefrigerationCyclePressureSpec.Pressure  cond_p_in_nominal=PlntThrCondNomPin Pa  cond_T_sat_nominal=400 K  cond_inlet_spec=fluids.two_phase_fluid.thermodynamic_cycles.enum.RefrigerationCycleInletSpec.Enthalpy  cond_T_in_nominal=PlntThrCondNomTin K  cond_h_in_nominal=500 kJ/kg  cond_x_in_nominal=1  cond_inlet_humidity_spec=foundation.enum.HumiditySpec.RelativeHumidity  cond_RH_in_nominal=PlntThrCondNomRelH  cond_x_w_in_nominal=0.01  cond_y_w_in_nominal=0.01  cond_HR_in_nominal=0.01  cond_Tw_in_nominal=287 K  cond_inlet_trace_gas_spec=foundation.enum.trace_gas_spec.mole_fraction  cond_x_g_in_nominal=cabin_CO2_init  cond_y_g_in_nominal=PlntThrCabCO2Init  cond_volume=PlntThrCycCondNomVol m^3  area_Ac=PlntThrCabDucArea m^2  area_Bc=PlntThrCabDucArea m^2  cond_wall_thermal_mass=true  cond_mass_wall=1 kg  cond_cp_wall=890 J/(K*kg)  cond_nominal_init=false  cond_p_init=EnvAbsPrs Pa  cond_energy_spec=foundation.enum.energy_spec.enthalpy  cond_T_init=EnvAirTemp K  cond_x_init=0.5  cond_alpha_init=0.5  cond_h_init=1500 kJ/kg  cond_u_init=1500 kJ/kg  cond_humidity_spec=foundation.enum.HumiditySpec.RelativeHumidity  cond_RH_init=PlntThrCabRelHInit  cond_x_w_init=0.01  cond_y_w_init=0.01  cond_HR_init=0.01  cond_Tw_init=287 K  cond_trace_gas_spec=foundation.enum.trace_gas_spec.mole_fraction  cond_x_g_init=0.001  cond_y_g_init=PlntThrCabCO2Init  cond_r_d_init=0  cond_T_wall_init=EnvAirTemp K  cond_RH_ws=1  cond_time_constant_cond=1e-3 s  cond_time_constant_evap=1e-3 s  cond_fraction_entrained=1  evap_domain=fluids.two_phase_fluid.thermodynamic_cycles.enum.RefrigerationCycleFluidDomain.ThermalLiquid  evap_mdot_nominal=PlntThrCycChlrH2OFlw kg/s  evap_delta_p_nominal=PlntThrCycChlrH2ODP Pa  evap_pressure_spec=fluids.two_phase_fluid.thermodynamic_cycles.enum.RefrigerationCyclePressureSpec.Pressure  evap_p_in_nominal=PlntThrCycChlrH2OPin Pa  evap_T_sat_nominal=400 K  evap_inlet_spec=fluids.two_phase_fluid.thermodynamic_cycles.enum.RefrigerationCycleInletSpec.Enthalpy  evap_T_in_nominal=PlntThrCycChlrH2OTin K  evap_h_in_nominal=500 kJ/kg  evap_x_in_nominal=1  evap_inlet_humidity_spec=foundation.enum.HumiditySpec.RelativeHumidity  evap_RH_in_nominal=0.1  evap_x_w_in_nominal=0.01  evap_y_w_in_nominal=0.01  evap_HR_in_nominal=0.01  evap_Tw_in_nominal=287 K  evap_inlet_trace_gas_spec=foundation.enum.trace_gas_spec.mass_fraction  evap_x_g_in_nominal=0.001  evap_y_g_in_nominal=0.001  evap_volume=PlntThrCycChlrH2OVol m^3  area_Ae=PlntThrPipeArea m^2  area_Be=PlntThrPipeArea m^2  evap_wall_thermal_mass=true  evap_mass_wall=1 kg  evap_cp_wall=890 J/(K*kg)  evap_nominal_init=false  evap_p_init=EnvAbsPrs Pa  evap_energy_spec=foundation.enum.energy_spec.enthalpy  evap_T_init=EnvAirTemp K  evap_x_init=0.5  evap_alpha_init=0.5  evap_h_init=1500 kJ/kg  evap_u_init=1500 kJ/kg  evap_humidity_spec=foundation.enum.HumiditySpec.RelativeHumidity  evap_RH_init=0.5  evap_x_w_init=0.01  evap_y_w_init=0.01  evap_HR_init=0.01  evap_Tw_init=287 K  evap_trace_gas_spec=foundation.enum.trace_gas_spec.mass_fraction  evap_x_g_init=0.001  evap_y_g_init=0.001  evap_r_d_init=0  evap_T_wall_init=EnvAirTemp K  evap_RH_ws=1  evap_time_constant_cond=1e-3 s  evap_time_constant_evap=1e-3 s  evap_fraction_entrained=1  cond_coeff_modify=false  cond_a_liq_refrig=0.023  cond_a_mix_refrig=0.005  cond_a_vap_refrig=0.023  cond_b_refrig=0.8  cond_c_refrig=0.33  cond_a_liq_extfld=0.023  cond_a_mix_extfld=0.005  cond_a_vap_extfld=0.023  cond_a_extfld=0.023  cond_b_extfld=0.8  cond_c_extfld=0.33  evap_coeff_modify=false  evap_a_liq_refrig=0.023  evap_a_mix_refrig=0.005  evap_a_vap_refrig=0.023  evap_b_refrig=0.8  evap_c_refrig=0.33  evap_a_liq_extfld=0.023  evap_a_mix_extfld=0.005  evap_a_vap_extfld=0.023  evap_a_extfld=0.023  evap_b_extfld=0.8  evap_c_extfld=0.33
      settings: InternalSimscapePortConfiguration="{\"Bottom\":[{\"id\":\"Ae_TL\",\"label\":\"Ae\",\"type\":\"foundation.thermal_liquid.thermal_liquid\"},{\"id\":\"Be_TL\",\"label\":\"Be\",\"type\":\"foundation.thermal_liquid.thermal_liquid\"}],\"Left\":[{\"id\":\"F\",\"label\":\"F\",\"type\":\"foundation.two_phase_fluid.two_phase_fluid\"},{\"id\":\"S\",\"label\":\"S\",\"type\":\"input\"}],\"Right\":[{\"id\":\"Qc\",\"label\":\"Qc\",\"type\":\"output\"},{\"id\":\"Qe\",\"label\":\"Qe\",\"type\":\"output\"},{\"id\":\"Pwr\",\"label\":\"Pwr\",\"type\":\"output\"},{\"id\":\"W\",\"label\":\"W\",\"type\":\"output\"}],\"Top\":[{\"id\":\"Ac_MA\",\"label\":\"Ac\",\"type\":\"foundation.moist_air.moist_air\"},{\"id\":\"Bc_MA\",\"label\":\"Bc\",\"type\":\"foundation.moist_air.moist_air\"}]}"
  Terminator{,1..3} (4 alike) : Terminator
  C : PMIOPort  Side=Left
  T : PMIOPort  Port=2  Side=Left
  D : PMIOPort  Port=3  Side=Right
  CondPress : Outport
  ChlrPress : Outport  Port=2
  CmpPwr : Outport  Port=3
  FanPwr : Outport  Port=4
  wires:
  PS-Simulink Converter/1 -> Terminator1/1
  PS-Simulink Converter1/1 -> Terminator/1
  CmpCmd/1 -> LPF with IC1/1(u)
  Probe Cycle/2 -> Terminator3/1
  Probe Cycle/1 -> Terminator2/1
  Probe Pressure/1 -> CondPress/1
  Probe Pressure/2 -> ChlrPress/1
  LPF with IC1/1(y) -> Simulink-PS Converter/1
  BaroPress/1 -> Environment/2(BaroPress)
  AmbTemp/1 -> Environment/1(AmbTemp)
  FanCmd/1 -> Environment/3(FanCmd)
  Environment/1(FanPwr) -> FanPwr/1
  PS-Simulink Converter2/1 -> CmpPwr/1
  connections:
  T/RConn1 -- System-Level Refrigeration Cycle (2P)/LConn3
  Refrigerant Properties/RConn1 -- System-Level Refrigeration Cycle (2P)/LConn1
  Environment/LConn1 -- System-Level Refrigeration Cycle (2P)/LConn4
  D/RConn1 -- System-Level Refrigeration Cycle (2P)/RConn6
  C/RConn1 -- System-Level Refrigeration Cycle (2P)/RConn5
  Simulink-PS Converter/RConn1 -- System-Level Refrigeration Cycle (2P)/LConn2
  PS-Simulink Converter/LConn1 -- System-Level Refrigeration Cycle (2P)/RConn2
  PS-Simulink Converter1/LConn1 -- System-Level Refrigeration Cycle (2P)/RConn1
  PS-Simulink Converter2/LConn1 -- System-Level Refrigeration Cycle (2P)/RConn3

== system ElectricalThermalSystemSSC/VEB Inputs/LPF with IC1 ==
  u : Inport
  Cont LPF IC : autolibutils/Cont LPF IC  wc=wc  aMode=1  dataType=off
  Initial Condition : Constant  Value=InitCond  SampleTime=-1
  y : Outport
  wires:
  Cont LPF IC/1 -> y/1
  u/1 -> Cont LPF IC/1
  Initial Condition/1 -> Cont LPF IC/2

== system ElectricalThermalSystemSSC/Motor/Cooling Assembly/CoolingAssy1 ==
  CoolEM1 : fl_lib/Thermal/Thermal Elements/Thermal Mass  mass_type=foundation.enum.constant_variable.constant  mass=1 kg  sp_heat=PlntEMCp J/kg/K  mass_min=1e-6 kg  num_ports=foundation.enum.numPorts2.two  m_specify=off  m_priority=High  m=1 kg  m_nominal_specify=off  m_nominal_value=1  m_nominal_unit=kg  T_specify=on  T_priority=High  T=EnvAirTemp K  T_nominal_specify=off  T_nominal_value=1  T_nominal_unit=K  Q_specify=off  Q_priority=None  Q=0 W  Q_nominal_specify=off  Q_nominal_value=1  Q_nominal_unit=W
      settings: InternalSimscapePortConfiguration="{\"Bottom\":[],\"Left\":[{\"id\":\"M\",\"label\":\"\",\"type\":\"foundation.thermal.thermal\"}],\"Right\":[{\"id\":\"N\",\"label\":\"\",\"type\":\"foundation.thermal.thermal\"}],\"Top\":[]}"
  Coolant Jacket : SimscapeFluids_lib/Thermal Liquid/Pipes & Fittings/Pipe (TL)  dynamic_compressibility=simscape.enum.onoff.on  inertia=simscape.enum.onoff.off  num_segments=1  pipe_length=PlntThrEMJacLen m  cross_section_geometry=fluids.thermal_liquid.pipes_fittings.enum.CrossSectionGeometry.Custom  pipe_diameter=0.1 m  pipe_inner_diameter=0.05 m  pipe_outer_diameter=0.1 m  pipe_width=0.1 m  pipe_height=0.1 m  pipe_major_axis=0.1 m  pipe_minor_axis=0.05 m  pipe_side=0.1 m  pipe_angle=30 deg  area=PlntThrChArea m^2  Dh=PlntThrChDia m  elevation_spec=foundation.enum.constant_variable.constant  elevation_gain=0 m  gravity_spec=foundation.enum.constant_variable.constant  g=EnvGrvty m/s^2  pressure_loss_spec=fluids.thermal_liquid.pipes_fittings.enum.PressureLossSpec.Haaland  local_pressure_loss_spec=fluids.thermal_liquid.pipes_fittings.enum.LocalLossSpec.AggregateLength  length_add=PlntThrEqLength m  loss_coefficient=0.1  roughness_spec=fluids.thermal_liquid.pipes_fittings.enum.RoughnessSpec.Custom  roughness=1.5e-5 m  Re_friction_TLU=[ 400 1000 1.5e+3 3e+3 4e+3 6e+3 1e+4 2e+4 4e+4 6e+4 1e+5 1e+8 ]  friction_factor_TLU=[ 0.264 0.112 0.07099999999999999 0.0417 0.0387 0.0268 0.025 0.0232 0.0226 0.022 0.0214 0.0214 ]  Re_lam=100  Re_tur=500  shape_factor=64  mdot_nominal=[ 0.1 1 ] kg/s  p_diff_nominal=[ 0.001 0.01 ] MPa  mdot_threshold=1e-6 kg/s  wall_spec=fluids.thermal_liquid.pipes_fittings.enum.wall_spec.rigid  vol_expansion_spec=fluids.thermal_liquid.pipes_fittings.enum.VolumeExpansionSpec.Diameter  area_pressure_gain=1e-6 m^2/MPa  static_pressure_TLU=[.1, 1] MPa  area_pressure_gain_TLU=[1e-05, 1.1e-05] m^2  material_behavior_spec=fluids.thermal_liquid.pipes_fittings.enum.PipeMaterialBehavior.Linear  diameter_pressure_gain=1.2e-6 m/MPa  wall_thickness=0.05 m  elastic_modulus=69 GPa  stress_TLU=[276, 310] MPa  strain_TLU=[.004, .02]  stress_assert_action=simscape.enum.assert.action.none  stress_max=400 MPa  poisson_ratio=0.33  wall_time_constant=0.01 s  thermal_expansion=false  alpha_L_wall=24 um/(deltaK*m)  thermal_expansion_Tref=293.15 K  heat_transfer_spec=fluids.thermal_liquid.pipes_fittings.enum.HeatTransferSpec.DittusBoelter  mdot_nominal_heat=[ 0.1 1 ] kg/s  T_in_nominal=[ 293.15 293.15 ] K  T_out_nominal=[ 300 300 ] K  p_in_nominal_heat=[ 0.101325 0.101325 ] MPa  T_wall_nominal=[ 303.15 303.15 ] K  a_coeff=0.3  b_Re_power=0.8  c_Pr_power=0.33  Nu_lam=3.66  Re_Colburn_TLU=[ 100 150 1000 ]  Colburn_factor_TLU=[ 0.019 0.013 0.002 ]  Re_Nu_TLU=[ 100 150 1000 ]  Pr_Nu_TLU=[ 1 10 ]  Nu_TLU=[ 3.72 4.21; 3.75 4.44; 4.21 7.15 ]  p0_vec=EnvAbsPrs Pa  T0_vec=EnvAirTemp K  mdot0=0.1 kg/s  p_nominal=0.101325 MPa  T_nominal=293.15 K
  Heat Flow Rate Sensor3 : fl_lib/Thermal/Thermal Sensors/Heat Flow Rate Sensor
  PS-Simulink Converter : nesl_utility/PS-Simulink Converter  PhysicalDomain=network_engine_domain  SubClassName=ps_output  LeftPortType=input  RightPortType=output  PseudoPeriodic=off  Frequencies=[]  VectorFormat=1-D array  Unit=K  AffineConversion=on
  PS-Simulink Converter4 : nesl_utility/PS-Simulink Converter  PhysicalDomain=network_engine_domain  SubClassName=ps_output  LeftPortType=input  RightPortType=output  PseudoPeriodic=off  Frequencies=[]  VectorFormat=inherit  Unit=W  AffineConversion=off
  Temperature Sensor : fl_lib/Thermal/Thermal Sensors/Temperature Sensor  temperature_measure=foundation.enum.MeasurementReference.difference
  Thermal Reference1 : fl_lib/Thermal/Thermal Elements/Thermal Reference
  H1 : PMIOPort  Side=Right
  A : PMIOPort  Port=2  Side=Left
  B : PMIOPort  Port=3  Side=Right
  EMTemp : Outport
  Qem : Outport  Port=2
  wires:
  PS-Simulink Converter4/1 -> Qem/1
  PS-Simulink Converter/1 -> EMTemp/1
  connections:
  PS-Simulink Converter4/LConn1 -- Heat Flow Rate Sensor3/RConn1
  Coolant Jacket/LConn2 -- Heat Flow Rate Sensor3/RConn2
  Heat Flow Rate Sensor3/LConn1 -- CoolEM1/RConn1 -- Temperature Sensor/LConn1
  CoolEM1/LConn1 -- H1/RConn1
  A/RConn1 -- Coolant Jacket/LConn1
  Coolant Jacket/RConn1 -- B/RConn1
  Temperature Sensor/RConn2 -- PS-Simulink Converter/LConn1
  Thermal Reference1/LConn1 -- Temperature Sensor/RConn1
